simulink model "TorqueVect_HIL_CAN"  (R2022a)
settings: Solver=VariableStepAuto  StartTime=0.0  StopTime=300  RelTol=1e-3
PreLoadFcn:
  | run('Parameters\FSE_Parameters.m')
values from neighbouring files (symbols this model uses):
  Kd = 0;')    [open_carmaker_gui.m]
  Ki = 0    [open_carmaker_gui.m]
undefined symbols (not defined in the file or in its folder): BRegenEnabledButton, canChannel, CyalphaLookUp, efficiency, Fz_curve, Fz_scaling_long, gearR, izz, jw, kd, ki, Kp, kp, l_f, l_r, lambda, m, Mz_max, N, N_lat, N_long, P_max, pid_kd_lat, pid_kd_long, pid_ki_lat, pid_ki_long, pid_kp_lat, pid_kp_long, R_max, rw, steerR, T_i_max, TC_Decr_Gas, TC_Derivative, TC_Incr_Gas, TC_On, TC_Relay_Off, TC_Relay_On, tireCornerStiffness, Ts, TV_On, TV_Override, velocity_lookup, velocity_lookup_lat, y_ref, yrr_scaling
libraries: simulink x218, slpidlib x135, CarMaker4SL x73, TractionControlLibrary x13, canmsglib x11, canlib x10, TorqueVectoringLibrary x6, simulink_extras x4, PedalConversionLibrary x3, PowerControlLibrary x1
(part 4 of 26)

== system TorqueVect_HIL_CAN/CarMaker/IPG Vehicle/PowerTrain/PTControl Example/PTControl_ALL_CTRL_VC_MFE24/New TC ==
  lim 1 : Inport
  lim 2 : Inport  Port=2
  lim 3 : Inport  Port=3
  lim 4 : Inport  Port=4
  vx : Inport  Port=5
  w_FL : Inport  Port=6
  w_FR : Inport  Port=7
  w_RL : Inport  Port=8
  w_RR : Inport  Port=9
  Front SR Target : Inport  Port=10
  Rear SR Target : Inport  Port=11
  P_TC : Inport  Port=12
  D_TC : Inport  Port=13
  enable_tc : Inport  Port=14
  rate_h : Inport  Port=15
  rate_l : Inport  Port=16
  Demux1 : Demux
  Gain : Gain  Gain=0.2032/13.39
  Rate Limiter Dynamic{,1..3} (4 alike) : simulink/Discontinuities/Rate Limiter Dynamic
  Reference Generator1 : Subsystem
  Saturation : Saturate  UpperLimit=inf  LowerLimit=0
  Subtract1 : Sum  Inputs=-+
  TC R1 : Subsystem
  TC R2 : Subsystem
  TC R3 : Subsystem
  TC R4 : Subsystem
  Vector Concatenate3 : Concatenate  NumInputs=4
  R1 Demand : Outport
  L1 Demand : Outport  Port=2
  R2 Demand : Outport  Port=3
  L2 Demand : Outport  Port=4
  wires:
  Reference Generator1/1(R1) -> TC R1/1(modified slip ratio reference)
  lim 1/1 -> TC R1/2(lim 1)
  Gain/1 -> Subtract1/2
  Vector Concatenate3/1 -> Gain/1  "omega"
  Subtract1/1 -> Demux1/1
  vx/1 -> Saturation/1
  TC R2/1(Control Effort 1) -> Rate Limiter Dynamic1/2  "MMotorL1Demand"
  w_RL/1 -> Vector Concatenate3/4
  w_RR/1 -> Vector Concatenate3/3
  w_FL/1 -> Vector Concatenate3/2
  w_FR/1 -> Vector Concatenate3/1
  Front SR Target/1 -> Reference Generator1/2(Front SR Target)
  Rear SR Target/1 -> Reference Generator1/3(Rear SR Target)
  lim 2/1 -> TC R2/2(lim 1)
  lim 3/1 -> TC R3/2(lim 1)
  lim 4/1 -> TC R4/2(lim 1)
  Reference Generator1/2(L1) -> TC R2/1(modified slip ratio reference)
  Reference Generator1/3(R2) -> TC R3/1(modified slip ratio reference)
  Reference Generator1/4(L2) -> TC R4/1(modified slip ratio reference)
  P_TC/1 -> TC R2/4(P_TC), TC R4/4(P_TC), TC R3/4(P_TC), TC R1/4(P_TC)
  D_TC/1 -> TC R2/5(D_TC), TC R4/5(D_TC), TC R3/5(D_TC), TC R1/5(D_TC)
  Demux1/1 -> TC R1/3(modified slip ratio measurement)
  Demux1/2 -> TC R2/3(modified slip ratio measurement)
  Demux1/3 -> TC R3/3(modified slip ratio measurement)
  Demux1/4 -> TC R4/3(modified slip ratio measurement)
  TC R1/1(Control Effort 1) -> Rate Limiter Dynamic/2  "MMotorR1Demand"
  Saturation/1 -> Subtract1/1, Reference Generator1/1(x2)
  TC R3/1(Control Effort 1) -> Rate Limiter Dynamic2/2
  TC R4/1(Control Effort 1) -> Rate Limiter Dynamic3/2
  enable_tc/1 -> TC R4/6(enable_tc), TC R2/6(enable_tc), TC R3/6(enable_tc), TC R1/6(enable_tc)
  Rate Limiter Dynamic/1 -> R1 Demand/1
  rate_h/1 -> Rate Limiter Dynamic3/1, Rate Limiter Dynamic2/1, Rate Limiter Dynamic1/1, Rate Limiter Dynamic/1
  rate_l/1 -> Rate Limiter Dynamic/3, Rate Limiter Dynamic3/3, Rate Limiter Dynamic2/3, Rate Limiter Dynamic1/3
  Rate Limiter Dynamic1/1 -> L1 Demand/1
  Rate Limiter Dynamic2/1 -> R2 Demand/1
  Rate Limiter Dynamic3/1 -> L2 Demand/1

== system TorqueVect_HIL_CAN/CarMaker/IPG Vehicle/PowerTrain/PTControl Example/PTControl_ALL_CTRL_VC_MFE24/PTC ==
  Constant2 : Constant
  Ground : Ground
  Mode_EngineDrive : Constant  Value=4
  Mux : Mux
  OperState_Driving : Constant  Value=4
  PTC MiscOut : Outport  VectorParamsAs1DForOutWhenUnconnected=off
  wires:
  Constant2/1 -> Mux/4  "Ignition"
  Mode_EngineDrive/1 -> Mux/3
  Ground/1 -> Mux/2  "OperationError"
  OperState_Driving/1 -> Mux/1
  Mux/1 -> PTC MiscOut/1

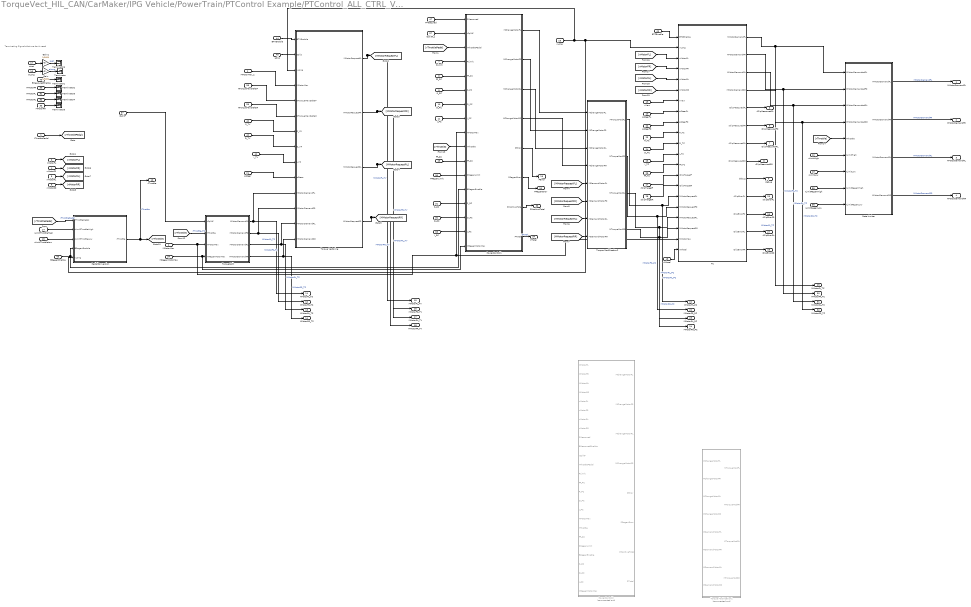
== system TorqueVect_HIL_CAN/CarMaker/IPG Vehicle/PowerTrain/PTControl Example/PTControl_ALL_CTRL_VC_MFE24/Subsystem ==
  note: Terminating Signals that we don't need
  rThrottlePedal : Inport
  MMotorMax : Inport  Port=2
  nMotorFL : Inport  Port=3
  nMotorFR : Inport  Port=4
  nMotorRL : Inport  Port=5
  nMotorRR : Inport  Port=6
  PLimit : Inport  Port=7
  FF_PC : Inport  Port=8
  P_PC : Inport  Port=9
  D_PC : Inport  Port=10
  I_PC : Inport  Port=11
  rLimitHigh : Inport  Port=12
  rLimitLow : Inport  Port=13
  rLimitThrottleHigh : Inport  Port=14
  rLimitThrottleLow : Inport  Port=15
  aLong : Inport  Port=16
  aLat : Inport  Port=17
  vLong : Inport  Port=18
  nYaw : Inport  Port=19
  aSteerFL : Inport  Port=20
  aSteer : Inport  Port=21
  aSteerFR : Inport  Port=22
  P_TC : Inport  Port=23
  D_TC : Inport  Port=24
  I_TC : Inport  Port=25
  FF_TC : Inport  Port=26
  rSlipTargetF : Inport  Port=27
  rSlipTargetR : Inport  Port=28
  FF_RC : Inport  Port=29
  PRegenLimit : Inport  Port=30
  P_RC : Inport  Port=31
  D_RC : Inport  Port=32
  I_RC : Inport  Port=33
  MRegenMotorMax : Inport  Port=34
  rLimitRegenHigh : Inport  Port=35
  rLimitRegenLow : Inport  Port=36
  rSplitF : Inport  Port=37
  NTorqueMaxDeltaF : Inport  Port=38
  NTorqueMaxDeltaR : Inport  Port=39
  P_TV : Inport  Port=40
  I_TV : Inport  Port=41
  D_TV : Inport  Port=42
  BRegenEnable : Inport  Port=43
  BTVEnable : Inport  Port=44
  aSlip : Inport  Port=45
  BTCEnable : Inport  Port=46
  PMeasured : Inport  Port=47  OutMin=-250000  OutMax=250000  Unit=W  PortDimensions=1
      settings: AttributesFormatString=[%<OutMin>, %<OutMax>] %<Unit>
  rWheel : Inport  Port=48
  BMeasuredEnable : Inport  Port=49
  MMotorFR : Inport  Port=50
  MMotorFL : Inport  Port=51
  MMotorRL : Inport  Port=52
  MMotorRR : Inport  Port=53
  Gain : Gain  Gain=1/9.81
  Gain1 : Gain  Gain=1/9.81
  MMotorMax_1 : InportShadow  Port=2
  PedalConversion : Subsystem
  PowerControl1 : Subsystem
  PowerControl2 : Subsystem  Commented=on
  Rate Limiter : Subsystem
  TC : Subsystem
  Terminator{,1..6} (7 alike) : Terminator
  Torque Modification1 : Subsystem  Commented=on
  Torque Modification2 : Subsystem
  Torque Vectoring : Subsystem
  TorqueSplit : Subsystem
  rSplitF_1 : InportShadow  Port=37
  MMotorDemandFL : Outport
  MMotorDemandFR : Outport  Port=2
  MMotorDemandRL : Outport  Port=3
  MMotorDemandRR : Outport  Port=4
  rSlipMeasuredFL : Outport  Port=5
  rSlipMeasuredFR : Outport  Port=6
  rSlipMeasuredRL : Outport  Port=7
  rSlipMeasuredRR : Outport  Port=8
  debug : Outport  Port=9
  rThrottle : Outport  Port=10
  MMotorFL_TS : Outport  Port=11
  MMotorFR_TS : Outport  Port=12
  MMotorRL_TS : Outport  Port=13
  MMotorRR_TS : Outport  Port=14
  MMotorFL_TV : Outport  Port=15
  MMotorFR_TV : Outport  Port=16
  MMotorRL_TV : Outport  Port=17
  MMotorRR_TV : Outport  Port=18
  PError : Outport  Port=19
  PRegenError : Outport  Port=20
  MMotorFL_PC : Outport  Port=21
  MMotorFR_PC : Outport  Port=22
  MMotorRL_PC : Outport  Port=23
  MMotorRR_PC : Outport  Port=24
  rSlipErrorFL : Outport  Port=25
  rSlipErrorFR : Outport  Port=26
  rSlipErrorRL : Outport  Port=27
  rSlipErrorRR : Outport  Port=28
  MMotorFL_TC : Outport  Port=29
  MMotorFR_TC : Outport  Port=30
  MMotorRL_TC : Outport  Port=31
  MMotorRR_TC : Outport  Port=32
  PPositiveTotal : Outport  Port=33
  PTotal : Outport  Port=34
  wires:
  nMotorFR/1 -> [nMotorFR]
  nMotorRR/1 -> [nMotorRR]
  rSlipTargetF/1 -> TC/14(rSlipTargetF)
  Torque Vectoring/1(MMotorRequestFL) -> MMotorFL_TV/1, [MMotorRequestFL]  "MMotorFL_TV"
  nMotorRL/1 -> [nMotorRL]
  P_RC/1 -> PowerControl1/14(P_RC)
  TC/2(MMotorDemandFR) -> MMotorFR_TC/1, Rate Limiter/2(MMotorDemandedFR)  "MMotorFR_TC"
  [nMotorFL] -> TC/3(nMotorFL)
  MRegenMotorMax/1 -> PowerControl1/17(MRegenMotorMax), TorqueSplit/4(MRegenMotorMax)
  Torque Vectoring/4(MMotorRequestRR) -> MMotorRR_TV/1, [MMotorRequestRR]  "MMotorRR_TV"
  PedalConversion/1(rThrottle) -> rThrottle/1, [rThrottle]  "rThrottle"
  rSlipTargetR/1 -> TC/15(rSlipTargetR)
  [rThrottle] -> TorqueSplit/2(rThrottle)  "rThrottle_TS"
  FF_PC/1 -> PowerControl1/5(FF_PC)
  aLong/1 -> Gain/1
  Torque Vectoring/2(MMotorRequestFR) -> MMotorFR_TV/1, [MMotorRequestFR]  "MMotorFR_TV"
  TC/1(MMotorDemandFL) -> MMotorFL_TC/1, Rate Limiter/1(MMotorDemandedFL)  "MMotorFL_TC"
  TC/10(rSlipErrorFL) -> rSlipErrorFL/1
  [rThrottle] -> Rate Limiter/5(rThrottle)
  rLimitThrottleHigh/1 -> PedalConversion/2(rLimitThrottleHigh)
  [MMotorRequestRL] -> Torque Modification2/7(MDemandMotorRL)
  TC/3(MMotorDemandRL) -> Rate Limiter/3(MMotorDemandedRL), MMotorRL_TC/1  "MMotorRL_TC"
  I_TC/1 -> TC/12(I_TC)
  TorqueSplit/2(MMotorDemandFR) -> MMotorFR_TS/1, Torque Vectoring/12(MMotorDemandFR)  "MMotorFR_TS"
  rLimitHigh/1 -> Rate Limiter/6(rLimitHigh)
  TC/5(rSlipMeasuredFL) -> rSlipMeasuredFL/1
  MMotorMax/1 -> PowerControl1/9(MMotorMax), TC/20(MMotorMax), TorqueSplit/3(MMotorMax)
  [nMotorRR] -> TC/6(nMotorRR)
  [rThrottle] -> PowerControl1/10(rThrottle)
  aSteerFR/1 -> TC/9(aSteerFR)
  Torque Vectoring/3(MMotorRequestRL) -> MMotorRL_TV/1, [MMotorRequestRL]  "MMotorRL_TV"
  rLimitRegenHigh/1 -> Rate Limiter/8(rLimitRegenHigh)
  P_TC/1 -> TC/10(P_TC)
  rSplitF/1 -> TorqueSplit/1(rSplitF)
  TorqueSplit/3(MMotorDemandRL) -> MMotorRL_TS/1, Torque Vectoring/13(MMotorDemandRL)  "MMotorRL_TS"
  [MMotorRequestRR] -> Torque Modification2/8(MDemandMotorRR)
  FF_TC/1 -> TC/13(FF_TC)
  P_PC/1 -> PowerControl1/6(P_PC)
  rLimitRegenLow/1 -> Rate Limiter/9(rLimitRegenLow)
  [MMotorRequestFL] -> Torque Modification2/5(MDemandMotorFL)
  [nMotorFR] -> TC/4(nMotorFR)
  rLimitLow/1 -> Rate Limiter/7(rLimitLow)
  D_TC/1 -> TC/11(D_TC)
  D_RC/1 -> PowerControl1/15(D_RC)
  vLong/1 -> Torque Vectoring/3(vLong), TC/2(vLong), PedalConversion/5(vLong)
  nYaw/1 -> TC/7(nYaw)
  TC/6(rSlipMeasuredFR) -> rSlipMeasuredFR/1
  PRegenLimit/1 -> PowerControl1/12(PRegenLimit)
  MMotorMax_1/1 -> Torque Vectoring/4(MMotorMax)
  rLimitThrottleLow/1 -> PedalConversion/3(rLimitThrottleLow)
  Rate Limiter/4(MMotorDemandRR) -> MMotorDemandRR/1  "MMotorDemandRR"
  nMotorFL/1 -> [nMotorFL]
  PLimit/1 -> PowerControl1/4(PLimit)
  Rate Limiter/3(MMotorDemandRL) -> MMotorDemandRL/1  "MMotorDemandRL"
  P_TV/1 -> Torque Vectoring/7(P_YR)
  rThrottlePedal/1 -> [rThrottlePedal]
  NTorqueMaxDeltaF/1 -> Torque Vectoring/5(NTorqueMaxDeltaF)
  rSplitF_1/1 -> PowerControl1/2(rSplitF)
  BTVEnable/1 -> Torque Vectoring/1(BTVEnable)
  TC/9(debug) -> debug/1
  D_TV/1 -> Torque Vectoring/8(D_YR)
  TC/7(rSlipMeasuredRL) -> rSlipMeasuredRL/1
  BTCEnable/1 -> TC/1(BTCEnable)
  [rThrottlePedal] -> PedalConversion/1(rThrottlePedal)  "rThrottlePedal"
  Rate Limiter/2(MMotorDemandFR) -> MMotorDemandFR/1  "MMotorDemandFR"
  TorqueSplit/1(MMotorDemandFL) -> MMotorFL_TS/1, Torque Vectoring/11(MMotorDemandFL)  "MMotorFL_TS"
  NTorqueMaxDeltaR/1 -> Torque Vectoring/6(NTorqueMaxDeltaR)
  TC/13(rSlipErrorRR) -> rSlipErrorRR/1
  aSteerFL/1 -> TC/8(aSteerFL)
  I_TV/1 -> Torque Vectoring/9(I_YR)
  TC/11(rSlipErrorFR) -> rSlipErrorFR/1
  I_RC/1 -> PowerControl1/16(I_RC)
  [MMotorRequestFR] -> Torque Modification2/6(MDemandMotorFR)
  [nMotorRL] -> TC/5(nMotorRL)
  aSlip/1 -> Torque Vectoring/2(aSlip)
  Rate Limiter/1(MMotorDemandFL) -> MMotorDemandFL/1  "MMotorDemandFL"
  I_PC/1 -> PowerControl1/8(I_PC)
  TC/4(MMotorDemandRR) -> MMotorRR_TC/1, Rate Limiter/4(MMotorDemandedRR)  "MMotorRR_TC"
  D_PC/1 -> PowerControl1/7(D_PC)
  [rThrottlePedal] -> PowerControl1/3(rThrottlePedal)
  TC/8(rSlipMeasuredRR) -> rSlipMeasuredRR/1
  BRegenEnable/1 -> PowerControl1/13(BRegenEnable), PedalConversion/4(BRegenEnable)
  TorqueSplit/4(MMotorDemandRR) -> MMotorRR_TS/1, Torque Vectoring/14(MMotorDemandRR)  "MMotorRR_TS"
  TC/12(rSlipErrorRL) -> rSlipErrorRL/1
  PMeasured/1 -> PowerControl1/1(PMeasured)
  rWheel/1 -> TC/21(rWheel)
  PowerControl1/5(PError) -> PError/1
  PowerControl1/6(PRegenError) -> PRegenError/1
  PowerControl1/7(PPositiveTotal) -> PPositiveTotal/1
  Torque Modification2/1(MTorqueModFL) -> MMotorFL_PC/1, TC/16(MMotorRequestFL)  "MMotorFL_PC"
  Torque Modification2/2(MTorqueModFR) -> MMotorFR_PC/1, TC/17(MMotorRequestFR)  "MMotorFR_PC"
  Torque Modification2/3(MTorqueModRL) -> TC/18(MMotorRequestRL), MMotorRL_PC/1  "MMotorRL_PC"
  Torque Modification2/4(MTorqueModRR) -> TC/19(MMotorRequestRR), MMotorRR_PC/1  "MMotorRR_PC"
  FF_RC/1 -> PowerControl1/11(FF_RC)
  BMeasuredEnable/1 -> Terminator1/1
  MMotorRR/1 -> Terminator5/1
  MMotorRL/1 -> Terminator4/1
  MMotorFL/1 -> Terminator3/1
  MMotorFR/1 -> Terminator2/1
  PowerControl1/8(PTotal) -> PTotal/1  "PTotal"
  PowerControl1/1(MChangeMotorFL) -> Torque Modification2/1(MChangeMotorFL)
  PowerControl1/2(MChangeMotorFR) -> Torque Modification2/2(MChangeMotorFR)
  PowerControl1/3(MChangeMotorRL) -> Torque Modification2/3(MChangeMotorRL)
  PowerControl1/4(MChangeMotorRR) -> Torque Modification2/4(MChangeMotorRR)
  Gain/1 -> Terminator/1  "aLong"
  aLat/1 -> Gain1/1
  Gain1/1 -> Terminator6/1  "aLat"
  aSteer/1 -> Torque Vectoring/10(aSteer)

== system TorqueVect_HIL_CAN/CarMaker/IPG Vehicle/PowerTrain/PTControl Example/PTControl_ALL_CTRL_VC_REGEN/New TC ==
  lim 1 : Inport
  lim 2 : Inport  Port=2
  lim 3 : Inport  Port=3
  lim 4 : Inport  Port=4
  vx : Inport  Port=5
  w_FL : Inport  Port=6
  w_FR : Inport  Port=7
  w_RL : Inport  Port=8
  w_RR : Inport  Port=9
  Front SR Target : Inport  Port=10
  Rear SR Target : Inport  Port=11
  P_TC : Inport  Port=12
  D_TC : Inport  Port=13
  enable_tc : Inport  Port=14
  rate_h : Inport  Port=15
  rate_l : Inport  Port=16
  Demux1 : Demux
  Gain : Gain  Gain=0.2032/13.39
  Rate Limiter Dynamic{,1..3} (4 alike) : simulink/Discontinuities/Rate Limiter Dynamic
  Reference Generator1 : Subsystem
  Saturation : Saturate  UpperLimit=inf  LowerLimit=0
  Subtract1 : Sum  Inputs=-+
  TC R1 : Subsystem
  TC R2 : Subsystem
  TC R3 : Subsystem
  TC R4 : Subsystem
  Vector Concatenate3 : Concatenate  NumInputs=4
  R1 Demand : Outport
  L1 Demand : Outport  Port=2
  R2 Demand : Outport  Port=3
  L2 Demand : Outport  Port=4
  wires:
  Reference Generator1/1(R1) -> TC R1/1(modified slip ratio reference)
  lim 1/1 -> TC R1/2(lim 1)
  Gain/1 -> Subtract1/2
  Vector Concatenate3/1 -> Gain/1  "omega"
  Subtract1/1 -> Demux1/1
  vx/1 -> Saturation/1
  TC R2/1(Control Effort 1) -> Rate Limiter Dynamic1/2  "MMotorL1Demand"
  w_RL/1 -> Vector Concatenate3/4
  w_RR/1 -> Vector Concatenate3/3
  w_FL/1 -> Vector Concatenate3/2
  w_FR/1 -> Vector Concatenate3/1
  Front SR Target/1 -> Reference Generator1/2(Front SR Target)
  Rear SR Target/1 -> Reference Generator1/3(Rear SR Target)
  lim 2/1 -> TC R2/2(lim 1)
  lim 3/1 -> TC R3/2(lim 1)
  lim 4/1 -> TC R4/2(lim 1)
  Reference Generator1/2(L1) -> TC R2/1(modified slip ratio reference)
  Reference Generator1/3(R2) -> TC R3/1(modified slip ratio reference)
  Reference Generator1/4(L2) -> TC R4/1(modified slip ratio reference)
  P_TC/1 -> TC R2/4(P_TC), TC R4/4(P_TC), TC R3/4(P_TC), TC R1/4(P_TC)
  D_TC/1 -> TC R2/5(D_TC), TC R4/5(D_TC), TC R3/5(D_TC), TC R1/5(D_TC)
  Demux1/1 -> TC R1/3(modified slip ratio measurement)
  Demux1/2 -> TC R2/3(modified slip ratio measurement)
  Demux1/3 -> TC R3/3(modified slip ratio measurement)
  Demux1/4 -> TC R4/3(modified slip ratio measurement)
  TC R1/1(Control Effort 1) -> Rate Limiter Dynamic/2  "MMotorR1Demand"
  Saturation/1 -> Subtract1/1, Reference Generator1/1(x2)
  TC R3/1(Control Effort 1) -> Rate Limiter Dynamic2/2
  TC R4/1(Control Effort 1) -> Rate Limiter Dynamic3/2
  enable_tc/1 -> TC R4/6(enable_tc), TC R2/6(enable_tc), TC R3/6(enable_tc), TC R1/6(enable_tc)
  Rate Limiter Dynamic/1 -> R1 Demand/1
  rate_h/1 -> Rate Limiter Dynamic3/1, Rate Limiter Dynamic2/1, Rate Limiter Dynamic1/1, Rate Limiter Dynamic/1
  rate_l/1 -> Rate Limiter Dynamic/3, Rate Limiter Dynamic3/3, Rate Limiter Dynamic2/3, Rate Limiter Dynamic1/3
  Rate Limiter Dynamic1/1 -> L1 Demand/1
  Rate Limiter Dynamic2/1 -> R2 Demand/1
  Rate Limiter Dynamic3/1 -> L2 Demand/1

== system TorqueVect_HIL_CAN/CarMaker/IPG Vehicle/PowerTrain/PTControl Example/PTControl_ALL_CTRL_VC_REGEN/PTC ==
  Constant2 : Constant
  Ground : Ground
  Mode_EngineDrive : Constant  Value=4
  Mux : Mux
  OperState_Driving : Constant  Value=4
  PTC MiscOut : Outport  VectorParamsAs1DForOutWhenUnconnected=off
  wires:
  Constant2/1 -> Mux/4  "Ignition"
  Mode_EngineDrive/1 -> Mux/3
  Ground/1 -> Mux/2  "OperationError"
  OperState_Driving/1 -> Mux/1
  Mux/1 -> PTC MiscOut/1

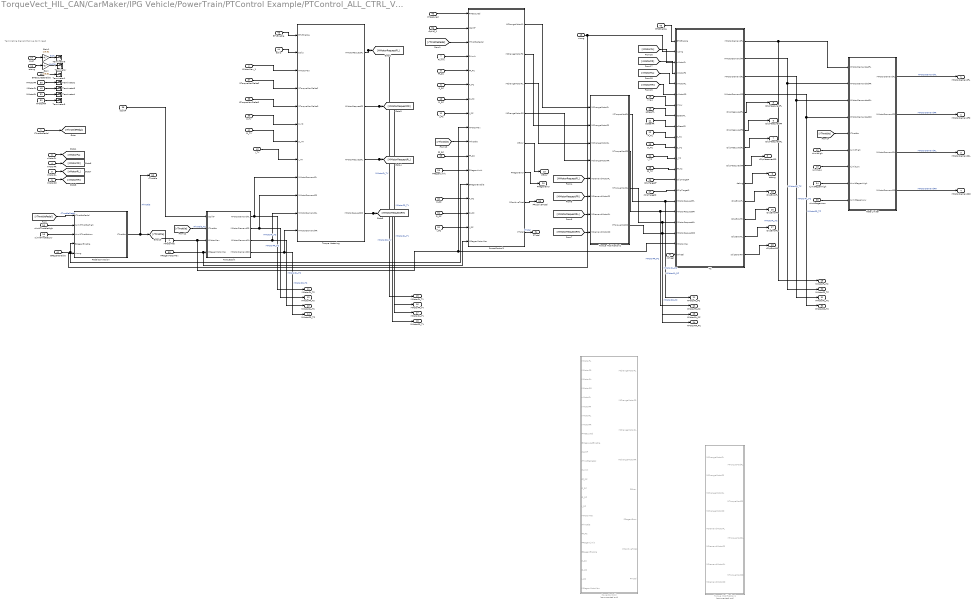
== system TorqueVect_HIL_CAN/CarMaker/IPG Vehicle/PowerTrain/PTControl Example/PTControl_ALL_CTRL_VC_REGEN/Subsystem ==
  note: Terminating Signals that we don't need
  rThrottlePedal : Inport
  MMotorMax : Inport  Port=2
  nMotorFL : Inport  Port=3
  nMotorFR : Inport  Port=4
  nMotorRL : Inport  Port=5
  nMotorRR : Inport  Port=6
  PLimit : Inport  Port=7
  FF_PC : Inport  Port=8
  P_PC : Inport  Port=9
  D_PC : Inport  Port=10
  I_PC : Inport  Port=11
  rLimitHigh : Inport  Port=12
  rLimitLow : Inport  Port=13
  rLimitThrottleHigh : Inport  Port=14
  rLimitThrottleLow : Inport  Port=15
  aLong : Inport  Port=16
  aLat : Inport  Port=17
  vLong : Inport  Port=18
  nYaw : Inport  Port=19
  aSteerFL : Inport  Port=20
  aSteerFR : Inport  Port=21
  P_TC : Inport  Port=22
  D_TC : Inport  Port=23
  I_TC : Inport  Port=24
  FF_TC : Inport  Port=25
  rSlipTargetF : Inport  Port=26
  rSlipTargetR : Inport  Port=27
  FF_RC : Inport  Port=28
  PRegenLimit : Inport  Port=29
  P_RC : Inport  Port=30
  D_RC : Inport  Port=31
  I_RC : Inport  Port=32
  MRegenMotorMax : Inport  Port=33
  rLimitRegenHigh : Inport  Port=34
  rLimitRegenLow : Inport  Port=35
  rSplitF : Inport  Port=36
  NTorqueMaxDeltaF : Inport  Port=37
  NTorqueMaxDeltaR : Inport  Port=38
  P_TV : Inport  Port=39
  I_TV : Inport  Port=40
  D_TV : Inport  Port=41
  BRegenEnable : Inport  Port=42
  BTVEnable : Inport  Port=43
  aSlip : Inport  Port=44
  BTCEnable : Inport  Port=45
  PMeasured : Inport  Port=46  OutMin=-250000  OutMax=250000  Unit=W  PortDimensions=1
      settings: AttributesFormatString=[%<OutMin>, %<OutMax>] %<Unit>
  rWheel : Inport  Port=47
  BMeasuredEnable : Inport  Port=48
  MMotorFL : Inport  Port=49
  MMotorFR : Inport  Port=50
  MMotorRL : Inport  Port=51
  MMotorRR : Inport  Port=52
  Gain : Gain  Gain=1/9.81
  Gain1 : Gain  Gain=1/9.81
  MMotorMax_1 : InportShadow  Port=2
  PedalConversion : Subsystem
  PowerControl1 : Subsystem
  PowerControl2 : Subsystem  Commented=on
  Rate Limiter : Subsystem
  TC : Subsystem
  Terminator{,1..6} (7 alike) : Terminator
  Torque Modification1 : Subsystem  Commented=on
  Torque Modification2 : Subsystem
  Torque Vectoring : Subsystem
  TorqueSplit : Subsystem
  rSplitF_1 : InportShadow  Port=36
  MMotorDemandFL : Outport
  MMotorDemandFR : Outport  Port=2
  MMotorDemandRL : Outport  Port=3
  MMotorDemandRR : Outport  Port=4
  rSlipMeasuredFL : Outport  Port=5
  rSlipMeasuredFR : Outport  Port=6
  rSlipMeasuredRL : Outport  Port=7
  rSlipMeasuredRR : Outport  Port=8
  debug : Outport  Port=9
  rThrottle : Outport  Port=10
  MMotorFL_TS : Outport  Port=11
  MMotorFR_TS : Outport  Port=12
  MMotorRL_TS : Outport  Port=13
  MMotorRR_TS : Outport  Port=14
  MMotorFL_TV : Outport  Port=15
  MMotorFR_TV : Outport  Port=16
  MMotorRL_TV : Outport  Port=17
  MMotorRR_TV : Outport  Port=18
  PError : Outport  Port=19
  PRegenError : Outport  Port=20
  MMotorFL_PC : Outport  Port=21
  MMotorFR_PC : Outport  Port=22
  MMotorRL_PC : Outport  Port=23
  MMotorRR_PC : Outport  Port=24
  rSlipErrorFL : Outport  Port=25
  rSlipErrorFR : Outport  Port=26
  rSlipErrorRL : Outport  Port=27
  rSlipErrorRR : Outport  Port=28
  MMotorFL_TC : Outport  Port=29
  MMotorFR_TC : Outport  Port=30
  MMotorRL_TC : Outport  Port=31
  MMotorRR_TC : Outport  Port=32
  PPositiveTotal : Outport  Port=33
  PTotal : Outport  Port=34
  wires:
  nMotorFR/1 -> [nMotorFR]
  nMotorRR/1 -> [nMotorRR]
  rSlipTargetF/1 -> TC/14(rSlipTargetF)
  Torque Vectoring/1(MMotorRequestFL) -> MMotorFL_TV/1, [MMotorRequestFL]  "MMotorFL_TV"
  nMotorRL/1 -> [nMotorRL]
  P_RC/1 -> PowerControl1/14(P_RC)
  TC/2(MMotorDemandFR) -> MMotorFR_TC/1, Rate Limiter/2(MMotorDemandedFR)  "MMotorFR_TC"
  [nMotorFL] -> TC/3(nMotorFL)
  MRegenMotorMax/1 -> PowerControl1/17(MRegenMotorMax), TorqueSplit/4(MRegenMotorMax)
  Torque Vectoring/4(MMotorRequestRR) -> MMotorRR_TV/1, [MMotorRequestRR]  "MMotorRR_TV"
  PedalConversion/1(rThrottle) -> rThrottle/1, [rThrottle]  "rThrottle"
  rSlipTargetR/1 -> TC/15(rSlipTargetR)
  [rThrottle] -> TorqueSplit/2(rThrottle)  "rThrottle_TS"
  FF_PC/1 -> PowerControl1/5(FF_PC)
  aLong/1 -> Gain/1
  Torque Vectoring/2(MMotorRequestFR) -> MMotorFR_TV/1, [MMotorRequestFR]  "MMotorFR_TV"
  TC/1(MMotorDemandFL) -> MMotorFL_TC/1, Rate Limiter/1(MMotorDemandedFL)  "MMotorFL_TC"
  TC/10(rSlipErrorFL) -> rSlipErrorFL/1
  [rThrottle] -> Rate Limiter/5(rThrottle)
  rLimitThrottleHigh/1 -> PedalConversion/2(rLimitThrottleHigh)
  [MMotorRequestRL] -> Torque Modification2/7(MDemandMotorRL)
  TC/3(MMotorDemandRL) -> Rate Limiter/3(MMotorDemandedRL), MMotorRL_TC/1  "MMotorRL_TC"
  I_TC/1 -> TC/12(I_TC)
  TorqueSplit/2(MMotorDemandFR) -> MMotorFR_TS/1, Torque Vectoring/10(MMotorDemandFR)  "MMotorFR_TS"
  rLimitHigh/1 -> Rate Limiter/6(rLimitHigh)
  TC/5(rSlipMeasuredFL) -> rSlipMeasuredFL/1
  MMotorMax/1 -> PowerControl1/9(MMotorMax), TC/20(MMotorMax), TorqueSplit/3(MMotorMax)
  [nMotorRR] -> TC/6(nMotorRR)
  [rThrottle] -> PowerControl1/10(rThrottle)
  aSteerFR/1 -> TC/9(aSteerFR)
  Torque Vectoring/3(MMotorRequestRL) -> MMotorRL_TV/1, [MMotorRequestRL]  "MMotorRL_TV"
  rLimitRegenHigh/1 -> Rate Limiter/8(rLimitRegenHigh)
  P_TC/1 -> TC/10(P_TC)
  rSplitF/1 -> TorqueSplit/1(rSplitF)
  TorqueSplit/3(MMotorDemandRL) -> MMotorRL_TS/1, Torque Vectoring/11(MMotorDemandRL)  "MMotorRL_TS"
  [MMotorRequestRR] -> Torque Modification2/8(MDemandMotorRR)
  FF_TC/1 -> TC/13(FF_TC)
  P_PC/1 -> PowerControl1/6(P_PC)
  rLimitRegenLow/1 -> Rate Limiter/9(rLimitRegenLow)
  [MMotorRequestFL] -> Torque Modification2/5(MDemandMotorFL)
  [nMotorFR] -> TC/4(nMotorFR)
  rLimitLow/1 -> Rate Limiter/7(rLimitLow)
  D_TC/1 -> TC/11(D_TC)
  D_RC/1 -> PowerControl1/15(D_RC)
  vLong/1 -> TC/2(vLong), PedalConversion/5(vLong)
  nYaw/1 -> TC/7(nYaw)
  TC/6(rSlipMeasuredFR) -> rSlipMeasuredFR/1
  PRegenLimit/1 -> PowerControl1/12(PRegenLimit)
  MMotorMax_1/1 -> Torque Vectoring/3(MMotorMax)
  rLimitThrottleLow/1 -> PedalConversion/3(rLimitThrottleLow)
  Rate Limiter/4(MMotorDemandRR) -> MMotorDemandRR/1  "MMotorDemandRR"
  nMotorFL/1 -> [nMotorFL]
  PLimit/1 -> PowerControl1/4(PLimit)
  Rate Limiter/3(MMotorDemandRL) -> MMotorDemandRL/1  "MMotorDemandRL"
  P_TV/1 -> Torque Vectoring/6(P_YR)
  rThrottlePedal/1 -> [rThrottlePedal]
  NTorqueMaxDeltaF/1 -> Torque Vectoring/4(NTorqueMaxDeltaF)
  rSplitF_1/1 -> PowerControl1/2(rSplitF)
  BTVEnable/1 -> Torque Vectoring/1(BTVEnable)
  TC/9(debug) -> debug/1
  D_TV/1 -> Torque Vectoring/7(D_YR)
  TC/7(rSlipMeasuredRL) -> rSlipMeasuredRL/1
  BTCEnable/1 -> TC/1(BTCEnable)
  [rThrottlePedal] -> PedalConversion/1(rThrottlePedal)  "rThrottlePedal"
  Rate Limiter/2(MMotorDemandFR) -> MMotorDemandFR/1  "MMotorDemandFR"
  TorqueSplit/1(MMotorDemandFL) -> MMotorFL_TS/1, Torque Vectoring/9(MMotorDemandFL)  "MMotorFL_TS"
  NTorqueMaxDeltaR/1 -> Torque Vectoring/5(NTorqueMaxDeltaR)
  TC/13(rSlipErrorRR) -> rSlipErrorRR/1
  aSteerFL/1 -> TC/8(aSteerFL)
  I_TV/1 -> Torque Vectoring/8(I_YR)
  TC/11(rSlipErrorFR) -> rSlipErrorFR/1
  I_RC/1 -> PowerControl1/16(I_RC)
  [MMotorRequestFR] -> Torque Modification2/6(MDemandMotorFR)
  [nMotorRL] -> TC/5(nMotorRL)
  aSlip/1 -> Torque Vectoring/2(aSlip)
  Rate Limiter/1(MMotorDemandFL) -> MMotorDemandFL/1  "MMotorDemandFL"
  I_PC/1 -> PowerControl1/8(I_PC)
  TC/4(MMotorDemandRR) -> MMotorRR_TC/1, Rate Limiter/4(MMotorDemandedRR)  "MMotorRR_TC"
  D_PC/1 -> PowerControl1/7(D_PC)
  [rThrottlePedal] -> PowerControl1/3(rThrottlePedal)
  TC/8(rSlipMeasuredRR) -> rSlipMeasuredRR/1
  BRegenEnable/1 -> PowerControl1/13(BRegenEnable), PedalConversion/4(BRegenEnable)
  TorqueSplit/4(MMotorDemandRR) -> MMotorRR_TS/1, Torque Vectoring/12(MMotorDemandRR)  "MMotorRR_TS"
  TC/12(rSlipErrorRL) -> rSlipErrorRL/1
  PMeasured/1 -> PowerControl1/1(PMeasured)
  rWheel/1 -> TC/21(rWheel)
  PowerControl1/5(PError) -> PError/1
  PowerControl1/6(PRegenError) -> PRegenError/1
  PowerControl1/7(PPositiveTotal) -> PPositiveTotal/1
  Torque Modification2/1(MTorqueModFL) -> MMotorFL_PC/1, TC/16(MMotorRequestFL)  "MMotorFL_PC"
  Torque Modification2/2(MTorqueModFR) -> MMotorFR_PC/1, TC/17(MMotorRequestFR)  "MMotorFR_PC"
  Torque Modification2/3(MTorqueModRL) -> TC/18(MMotorRequestRL), MMotorRL_PC/1  "MMotorRL_PC"
  Torque Modification2/4(MTorqueModRR) -> TC/19(MMotorRequestRR), MMotorRR_PC/1  "MMotorRR_PC"
  FF_RC/1 -> PowerControl1/11(FF_RC)
  BMeasuredEnable/1 -> Terminator1/1
  MMotorRR/1 -> Terminator5/1
  MMotorRL/1 -> Terminator4/1
  MMotorFL/1 -> Terminator3/1
  MMotorFR/1 -> Terminator2/1
  PowerControl1/8(PTotal) -> PTotal/1  "PTotal"
  PowerControl1/1(MChangeMotorFL) -> Torque Modification2/1(MChangeMotorFL)
  PowerControl1/2(MChangeMotorFR) -> Torque Modification2/2(MChangeMotorFR)
  PowerControl1/3(MChangeMotorRL) -> Torque Modification2/3(MChangeMotorRL)
  PowerControl1/4(MChangeMotorRR) -> Torque Modification2/4(MChangeMotorRR)
  Gain/1 -> Terminator/1  "aLong"
  aLat/1 -> Gain1/1
  Gain1/1 -> Terminator6/1  "aLat"

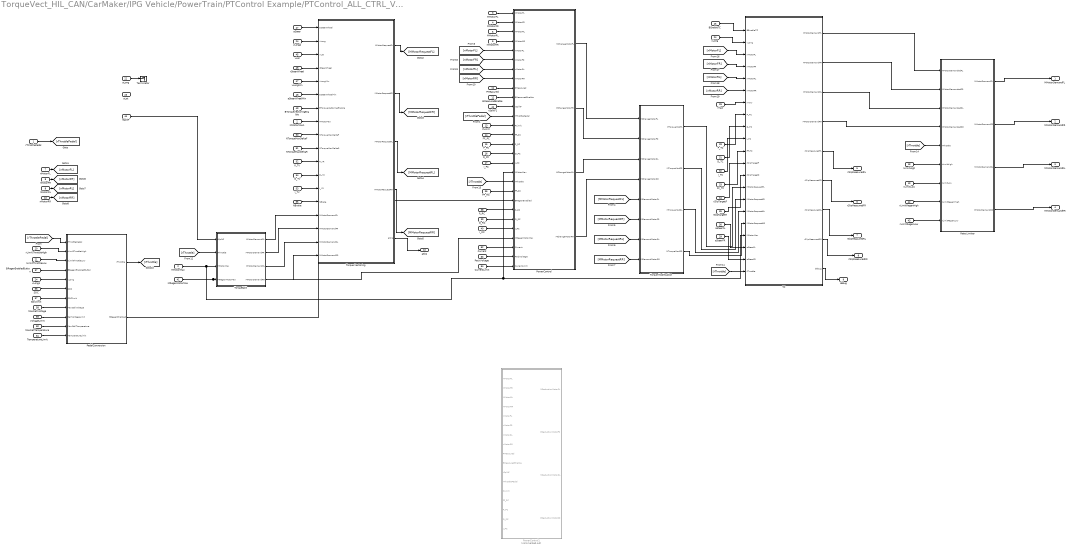
== system TorqueVect_HIL_CAN/CarMaker/IPG Vehicle/PowerTrain/PTControl Example/PTControl_ALL_CTRL_VC_REGEN/Subsystem1 ==
  rThrottlePedal : Inport
  MMotorMax : Inport  Port=2
  MMotorFL : Inport  Port=3
  MMotorFR : Inport  Port=4
  MMotorRL : Inport  Port=5
  MMotorRR : Inport  Port=6
  nMotorFL : Inport  Port=7
  nMotorFR : Inport  Port=8
  nMotorRL : Inport  Port=9
  nMotorRR : Inport  Port=10
  PMeasured : Inport  Port=11
  BMeasuredEnable : Inport  Port=12
  PLimit : Inport  Port=13
  FF_PC : Inport  Port=14
  P_PC : Inport  Port=15
  D_PC : Inport  Port=16
  I_PC : Inport  Port=17
  rLimitHigh : Inport  Port=18
  rLimitLow : Inport  Port=19
  rLimitThrottleHigh : Inport  Port=20
  rLimitThrottleLow : Inport  Port=21
  aLong : Inport  Port=22
  aLat : Inport  Port=23
  vLong : Inport  Port=24
  BEnableTC : Inport  Port=25
  nYaw : Inport  Port=26
  aSteer : Inport  Port=27
  P_TC : Inport  Port=28
  aSteerFR : Inport  Port=29
  aSteerFL : Inport  Port=30
  D_TC : Inport  Port=31
  I_TC : Inport  Port=32
  FF_TC : Inport  Port=33
  rSlipTargetF : Inport  Port=34
  rSlipTargetR : Inport  Port=35
  FF_RC : Inport  Port=36
  BRegenEnabledButton : Inport  Port=37
  P_RC : Inport  Port=38
  D_RC : Inport  Port=39
  I_RC : Inport  Port=40
  MRegenMotorMax : Inport  Port=41
  rLimitRegenHigh : Inport  Port=42
  rLimitRegenLow : Inport  Port=43
  rSplitF : Inport  Port=44
  vLat : Inport  Port=45
  rSteerWheel : Inport  Port=46
  vLongMin : Inport  Port=47
  aSteerWheelMin : Inport  Port=48
  BTorqueVectoringEnable : Inport  Port=49
  NTorqueMaxDeltaF : Inport  Port=50
  NTorqueMaxDeltaR : Inport  Port=51
  P_TV : Inport  Port=52
  I_TV : Inport  Port=53
  D_TV : Inport  Port=54
  NBrake : Inport  Port=55
  SOC : Inport  Port=56
  SOClimit : Inport  Port=57
  MaxCellVoltage : Inport  Port=58
  VoltageLimit : Inport  Port=59
  MaxCellTemperature : Inport  Port=60
  TemperatureLimit : Inport  Port=61
  Current : Inport  Port=62
  PackVoltage : Inport  Port=63
  CurrentLimit : Inport  Port=64
  MMotorMax1 : InportShadow  Port=2
  PedalConversion : Subsystem
  PowerControl : Subsystem
  PowerControl1 : Subsystem  Commented=on
  Rate Limiter : Subsystem
  TC : Subsystem
  Terminator : Terminator
  Torque Modification : Subsystem
  Torque Vectoring : Subsystem
  TorqueSplit : Subsystem
  rSplitF1 : InportShadow  Port=44
  vLong1 : InportShadow  Port=24
  vLong2 : InportShadow  Port=24
  MMotorDemandFL : Outport
  MMotorDemandFR : Outport  Port=2
  MMotorDemandRL : Outport  Port=3
  MMotorDemandRR : Outport  Port=4
  rSlipMeasuredFL : Outport  Port=5
  rSlipMeasuredFR : Outport  Port=6
  rSlipMeasuredRL : Outport  Port=7
  rSlipMeasuredRR : Outport  Port=8
  debug : Outport  Port=9
  aSlip : Outport  Port=10
  wires:
  FF_PC/1 -> PowerControl/14(FF_PC)
  MMotorFR/1 -> PowerControl/2(MMotorFR)
  P_PC/1 -> PowerControl/15(P_PC)
  rThrottlePedal/1 -> [rThrottlePedal]
  MMotorFL/1 -> PowerControl/1(MMotorFL)
  PLimit/1 -> PowerControl/13(PLimit)
  PedalConversion/1(rThrottle) -> [rThrottle]
  D_PC/1 -> PowerControl/16(D_PC)
  [rThrottlePedal] -> PowerControl/12(rThrottlePedal)
  I_PC/1 -> PowerControl/17(I_PC)
  MMotorRR/1 -> PowerControl/4(MMotorRR)
  MMotorRL/1 -> PowerControl/3(MMotorRL)
  PMeasured/1 -> PowerControl/9(PMeasured)
  BMeasuredEnable/1 -> PowerControl/10(BMeasuredEnable)
  [rThrottlePedal] -> PedalConversion/1(rThrottlePedal)
  Rate Limiter/1(MMotorDemandFL) -> MMotorDemandFL/1
  Rate Limiter/2(MMotorDemandFR) -> MMotorDemandFR/1
  Rate Limiter/3(MMotorDemandRL) -> MMotorDemandRL/1
  Rate Limiter/4(MMotorDemandRR) -> MMotorDemandRR/1
  rLimitHigh/1 -> Rate Limiter/6(rLimitHigh)
  rSplitF/1 -> TorqueSplit/1(rSplitF)
  MMotorMax/1 -> TC/18(MMotorMax), PowerControl/18(MMotorMax), TorqueSplit/3(MMotorMax)
  rLimitThrottleHigh/1 -> PedalConversion/2(rLimitThrottleHigh)
  rLimitThrottleLow/1 -> PedalConversion/3(rLimitThrottleLow)
  [nMotorFR] -> TC/4(nMotorFR)
  [nMotorFL] -> TC/3(nMotorFL)
  [nMotorRL] -> TC/5(nMotorRL)
  rSlipTargetR/1 -> TC/13(rSlipTargetR)
  P_TC/1 -> TC/8(P_TC)
  rSlipTargetF/1 -> TC/12(rSlipTargetF)
  [nMotorRR] -> TC/6(nMotorRR)
  BEnableTC/1 -> TC/1(BEnableTC)
  I_TC/1 -> TC/10(I_TC)
  D_TC/1 -> TC/9(D_TC)
  FF_TC/1 -> TC/11(FF_TC)
  nYaw/1 -> TC/7(nYaw)
  nMotorFL/1 -> [nMotorFL]
  nMotorFR/1 -> [nMotorFR]
  nMotorRL/1 -> [nMotorRL]
  nMotorRR/1 -> [nMotorRR]
  [nMotorRR] -> PowerControl/8(nMotorRR)
  [nMotorRL] -> PowerControl/7(nMotorRL)
  [nMotorFR] -> PowerControl/6(nMotorFR)
  [nMotorFL] -> PowerControl/5(nMotorFL)
  PowerControl/1(MChangeMotorFL) -> Torque Modification/1(MChangeMotorFL)
  PowerControl/2(MChangeMotorFR) -> Torque Modification/2(MChangeMotorFR)
  PowerControl/3(MChangeMotorRL) -> Torque Modification/3(MChangeMotorRL)
  PowerControl/4(MChangeMotorRR) -> Torque Modification/4(MChangeMotorRR)
  [MMotorRequestFL] -> Torque Modification/5(MDemandMotorFL)
  [MMotorRequestFR] -> Torque Modification/6(MDemandMotorFR)
  [MMotorRequestRL] -> Torque Modification/7(MDemandMotorRL)
  [MMotorRequestRR] -> Torque Modification/8(MDemandMotorRR)
  Torque Modification/4(MTorqueModRR) -> TC/17(MMotorRequestRR)
  Torque Modification/3(MTorqueModRL) -> TC/16(MMotorRequestRL)
  Torque Modification/2(MTorqueModFR) -> TC/15(MMotorRequestFR)
  Torque Modification/1(MTorqueModFL) -> TC/14(MMotorRequestFL)
  TC/1(MMotorDemandFL) -> Rate Limiter/1(MMotorDemandedFL)
  TC/2(MMotorDemandFR) -> Rate Limiter/2(MMotorDemandedFR)
  TC/3(MMotorDemandRL) -> Rate Limiter/3(MMotorDemandedRL)
  TC/4(MMotorDemandRR) -> Rate Limiter/4(MMotorDemandedRR)
  aLong/1 -> Terminator/1
  TC/5(rSlipMeasuredFL) -> rSlipMeasuredFL/1
  TC/6(rSlipMeasuredFR) -> rSlipMeasuredFR/1
  TC/7(rSlipMeasuredRL) -> rSlipMeasuredRL/1
  TC/8(rSlipMeasuredRR) -> rSlipMeasuredRR/1
  TC/9(debug) -> debug/1
  FF_RC/1 -> PowerControl/20(FF_RC)
  vLong1/1 -> PedalConversion/5(vLong)
  BRegenEnabledButton/1 -> PedalConversion/4(BRegenEnabledButton)
  P_RC/1 -> PowerControl/22(P_RC)
  D_RC/1 -> PowerControl/23(D_RC)
  I_RC/1 -> PowerControl/24(I_RC)
  MRegenMotorMax/1 -> PowerControl/25(MRegenMotorMax), TorqueSplit/4(MRegenMotorMax)
  [rThrottle] -> TorqueSplit/2(rThrottle)
  [rThrottle] -> PowerControl/19(rThrottle)
  [rThrottle] -> Rate Limiter/5(rThrottle)
  rLimitRegenHigh/1 -> Rate Limiter/8(rLimitRegenHigh)
  vLong/1 -> TC/2(vLong)
  rLimitLow/1 -> Rate Limiter/7(rLimitLow)
  rLimitRegenLow/1 -> Rate Limiter/9(rLimitRegenLow)
  Torque Vectoring/1(MMotorRequestFL) -> [MMotorRequestFL]
  Torque Vectoring/2(MMotorRequestFR) -> [MMotorRequestFR]
  Torque Vectoring/3(MMotorRequestRL) -> [MMotorRequestRL]
  Torque Vectoring/4(MMotorRequestRR) -> [MMotorRequestRR]
  TorqueSplit/1(MMotorDemandFL) -> Torque Vectoring/15(MMotorDemandFL)
  TorqueSplit/2(MMotorDemandFR) -> Torque Vectoring/16(MMotorDemandFR)
  TorqueSplit/3(MMotorDemandRL) -> Torque Vectoring/17(MMotorDemandRL)
  TorqueSplit/4(MMotorDemandRR) -> Torque Vectoring/18(MMotorDemandRR)
  aSteer/1 -> Torque Vectoring/1(aSteerWheel)
  vLong2/1 -> Torque Vectoring/2(vLong)
  vLat/1 -> Torque Vectoring/3(vLat)
  rSteerWheel/1 -> Torque Vectoring/4(rSteerWheel)
  vLongMin/1 -> Torque Vectoring/5(vLongMin)
  aSteerWheelMin/1 -> Torque Vectoring/6(aSteerWheelMin)
  BTorqueVectoringEnable/1 -> Torque Vectoring/7(BTorqueVectoringEnable)
  MMotorMax1/1 -> Torque Vectoring/8(MMotorMax)
  NTorqueMaxDeltaF/1 -> Torque Vectoring/9(NTorqueMaxDeltaF)
  NTorqueMaxDeltaR/1 -> Torque Vectoring/10(NTorqueMaxDeltaR)
  P_TV/1 -> Torque Vectoring/11(P_YR)
  I_TV/1 -> Torque Vectoring/13(I_YR)
  D_TV/1 -> Torque Vectoring/12(D_YR)
  NBrake/1 -> Torque Vectoring/14(NBrake)
  rSplitF1/1 -> PowerControl/11(rSplitF)
  PedalConversion/2(BRegenEnabled) -> PowerControl/21(BRegenEnabled)
  SOC/1 -> PedalConversion/6(SOC)
  SOClimit/1 -> PedalConversion/7(SOClimit)
  TemperatureLimit/1 -> PedalConversion/11(TemperatureLimit)
  MaxCellVoltage/1 -> PedalConversion/8(MaxCellVoltage)
  MaxCellTemperature/1 -> PedalConversion/10(MaxCellTemperature)
  VoltageLimit/1 -> PedalConversion/9(CellVoltageLimit)
  PackVoltage/1 -> PowerControl/27(PackVoltage)
  Current/1 -> PowerControl/26(Current)
  CurrentLimit/1 -> PowerControl/28(CurrentLimit)
  Torque Vectoring/5(aSlip) -> aSlip/1
  [rThrottle] -> TC/21(rThrottle)
  aSteerFL/1 -> TC/19(aSteerFL)
  aSteerFR/1 -> TC/20(aSteerFR)

== system TorqueVect_HIL_CAN/CarMaker/IPG Vehicle/PowerTrain/PTControl Example/PTControl_ALL_Speedgoat/New TC ==
  lim 1 : Inport
  lim 2 : Inport  Port=2
  lim 3 : Inport  Port=3
  lim 4 : Inport  Port=4
  vx : Inport  Port=5
  w_FL : Inport  Port=6
  w_FR : Inport  Port=7
  w_RL : Inport  Port=8
  w_RR : Inport  Port=9
  Front SR Target : Inport  Port=10
  Rear SR Target : Inport  Port=11
  P_TC : Inport  Port=12
  D_TC : Inport  Port=13
  enable_tc : Inport  Port=14
  rate_h : Inport  Port=15
  rate_l : Inport  Port=16
  Demux1 : Demux
  Gain : Gain  Gain=0.2032/13.39
  Rate Limiter Dynamic{,1..3} (4 alike) : simulink/Discontinuities/Rate Limiter Dynamic
  Reference Generator1 : Subsystem
  Saturation : Saturate  UpperLimit=inf  LowerLimit=0
  Subtract1 : Sum  Inputs=-+
  TC R1 : Subsystem
  TC R2 : Subsystem
  TC R3 : Subsystem
  TC R4 : Subsystem
  Vector Concatenate3 : Concatenate  NumInputs=4
  R1 Demand : Outport
  L1 Demand : Outport  Port=2
  R2 Demand : Outport  Port=3
  L2 Demand : Outport  Port=4
  wires:
  Reference Generator1/1(R1) -> TC R1/1(modified slip ratio reference)
  lim 1/1 -> TC R1/2(lim 1)
  Gain/1 -> Subtract1/2
  Vector Concatenate3/1 -> Gain/1  "omega"
  Subtract1/1 -> Demux1/1
  vx/1 -> Saturation/1
  TC R2/1(Control Effort 1) -> Rate Limiter Dynamic1/2  "MMotorL1Demand"
  w_RL/1 -> Vector Concatenate3/4
  w_RR/1 -> Vector Concatenate3/3
  w_FL/1 -> Vector Concatenate3/2
  w_FR/1 -> Vector Concatenate3/1
  Front SR Target/1 -> Reference Generator1/2(Front SR Target)
  Rear SR Target/1 -> Reference Generator1/3(Rear SR Target)
  lim 2/1 -> TC R2/2(lim 1)
  lim 3/1 -> TC R3/2(lim 1)
  lim 4/1 -> TC R4/2(lim 1)
  Reference Generator1/2(L1) -> TC R2/1(modified slip ratio reference)
  Reference Generator1/3(R2) -> TC R3/1(modified slip ratio reference)
  Reference Generator1/4(L2) -> TC R4/1(modified slip ratio reference)
  P_TC/1 -> TC R2/4(P_TC), TC R4/4(P_TC), TC R3/4(P_TC), TC R1/4(P_TC)
  D_TC/1 -> TC R2/5(D_TC), TC R4/5(D_TC), TC R3/5(D_TC), TC R1/5(D_TC)
  Demux1/1 -> TC R1/3(modified slip ratio measurement)
  Demux1/2 -> TC R2/3(modified slip ratio measurement)
  Demux1/3 -> TC R3/3(modified slip ratio measurement)
  Demux1/4 -> TC R4/3(modified slip ratio measurement)
  TC R1/1(Control Effort 1) -> Rate Limiter Dynamic/2  "MMotorR1Demand"
  Saturation/1 -> Subtract1/1, Reference Generator1/1(x2)
  TC R3/1(Control Effort 1) -> Rate Limiter Dynamic2/2
  TC R4/1(Control Effort 1) -> Rate Limiter Dynamic3/2
  enable_tc/1 -> TC R4/6(enable_tc), TC R2/6(enable_tc), TC R3/6(enable_tc), TC R1/6(enable_tc)
  Rate Limiter Dynamic/1 -> R1 Demand/1
  rate_h/1 -> Rate Limiter Dynamic3/1, Rate Limiter Dynamic2/1, Rate Limiter Dynamic1/1, Rate Limiter Dynamic/1
  rate_l/1 -> Rate Limiter Dynamic/3, Rate Limiter Dynamic3/3, Rate Limiter Dynamic2/3, Rate Limiter Dynamic1/3
  Rate Limiter Dynamic1/1 -> L1 Demand/1
  Rate Limiter Dynamic2/1 -> R2 Demand/1
  Rate Limiter Dynamic3/1 -> L2 Demand/1

== system TorqueVect_HIL_CAN/CarMaker/IPG Vehicle/PowerTrain/PTControl Example/PTControl_ALL_Speedgoat/PTC ==
  Constant2 : Constant
  Ground : Ground
  Mode_EngineDrive : Constant  Value=4
  Mux : Mux
  OperState_Driving : Constant  Value=4
  PTC MiscOut : Outport  VectorParamsAs1DForOutWhenUnconnected=off
  wires:
  Constant2/1 -> Mux/4  "Ignition"
  Mode_EngineDrive/1 -> Mux/3
  Ground/1 -> Mux/2  "OperationError"
  OperState_Driving/1 -> Mux/1
  Mux/1 -> PTC MiscOut/1

== system TorqueVect_HIL_CAN/CarMaker/IPG Vehicle/PowerTrain/PTControl Example/PTControl_ALL_Speedgoat/Subsystem ==
  VhclCtrl.PT : Inport
  PTControl_In : Inport  Port=2
  Bus Selector : BusSelector  OutputSignals=VhclCtrl Gas,VhclCtrl Brake
  Bus Selector1 : BusSelector  OutputSignals=Vel_B x,Vel_B y,Omega_B z,Acc_B x,Acc_B y
  Bus Selector2 : BusSelector  OutputSignals=PT:Motor.PT:Motor:Trq,PT:Motor.PT:Motor1:Trq,PT:Motor.PT:Motor2:Trq,PT:Motor.PT:Motor3:Trq,PT:Motor.PT:Motor:rotv,PT:Motor.PT:Motor1:rotv,PT:Motor.PT:Motor2:rotv,PT:Motor.PT:Motor3:rotv,Steer.Driver:Steer:Ang,Steer.Car:SteerAngle:FL,Steer.Car:SteerAngle:FR,PT:PwrSupply:HV1:Pwr
  CAN Configuration : canlib/CAN Configuration  BlockHandle=5539.0005  Device=MathWorks Virtual 1 (Channel 1)  DeviceMenu=MathWorks Virtual 1 (Channel 1)  ObjConstructor=canChannel('MathWorks', 'Virtual 1', 1)  BusSpeed=500000  EnableBitParameters=off  AckMode=Normal
      settings: SourceProductBaseCode=VN
  CAN Pack1 : canmsglib/CAN Pack  MsgList=(none)  MsgName=Wheel Torques  MsgIDType=Standard (11-bit identifier)  MsgIdentifier=600  MsgLength=8  Remote=off  ApplyMinMax=off  BusOutput=off  SignalInfo={ 'FL_Trq', '0', '16', 'LE', 'signed', 'Standard', '0', '1', '0', '-210', '210'; 'FR_Trq', '16', '16', 'LE', 'signed', 'Standard', '0', '1', '0', '-210', '210'; 'RL_Trq', '32', '16', 'LE', 'signed', 'Standard', '0', '1', '0', '-210', '210'; 'RR_Trq', '48', '16', 'LE', 'signed', 'Standard', '0', '1', '0', '-210', '210' }
      settings: SourceProductBaseCode=XP,ME,VN  DataFormat=manually specified signals
  CAN Pack2 : canmsglib/CAN Pack  MsgList=(none)  MsgName=Motor Speeds (rad/s)  MsgIDType=Standard (11-bit identifier)  MsgIdentifier=601  MsgLength=8  Remote=off  ApplyMinMax=off  BusOutput=off  SignalInfo={ 'FL_w', '0', '16', 'LE', 'signed', 'Standard', '0', '1', '0', '-32768', '32767'; 'FR_w', '16', '16', 'LE', 'signed', 'Standard', '0', '1', '0', '-32768', '32767'; 'RL_w', '32', '16', 'LE', 'signed', 'Standard', '0', '1', '0', '-32768', '32767'; 'RR_w', '48', '16', 'LE', 'signed', 'Standard', '0', '1', '0', '-32768', '32767' }
      settings: SourceProductBaseCode=XP,ME,VN  DataFormat=manually specified signals
  CAN Pack3 : canmsglib/CAN Pack  MsgList=(none)  MsgName=CAN Msg  MsgIDType=Standard (11-bit identifier)  MsgIdentifier=602  MsgLength=8  Remote=off  ApplyMinMax=off  BusOutput=off  SignalInfo={ 'Throttle', '0', '8', 'LE', 'unsigned', 'Standard', '0', '1', '0', '0', '100'; 'Brake', '8', '8', 'LE', 'unsigned', 'Standard', '0', '1', '0', '0', '100'; 'Steering Angle', '16', '16', 'LE', 'signed', 'Standard', '0', '1', '0', '-32768', '32767'; 'FL Angle', '32', '16', 'LE', 'signed', 'Standard', '0', '1', '0', '-32768', '32767'; 'FR Angle', '48', '16', 'LE', 'signed', 'Standard', '0', '1', '0', '-32768', '32767' }
      settings: SourceProductBaseCode=XP,ME,VN  DataFormat=manually specified signals
  CAN Pack4 : canmsglib/CAN Pack  MsgList=(none)  MsgName=CAN Msg  MsgIDType=Standard (11-bit identifier)  MsgIdentifier=603  MsgLength=8  Remote=off  ApplyMinMax=off  BusOutput=off  SignalInfo={ 'Vx', '0', '16', 'LE', 'signed', 'Standard', '0', '1', '0', '-32768', '32767'; 'Vy', '16', '16', 'LE', 'signed', 'Standard', '0', '1', '0', '-32768', '32767'; 'nYaw', '32', '16', 'LE', 'signed', 'Standard', '0', '1', '0', '-32768', '32767'; 'Power', '48', '16', 'LE', 'signed', 'Standard', '0', '1', '0', '-8000', '8000' }
      settings: SourceProductBaseCode=XP,ME,VN  DataFormat=manually specified signals
  CAN Pack5 : canmsglib/CAN Pack  Commented=on  MsgList=(none)  MsgName=CAN Msg  MsgIDType=Standard (11-bit identifier)  MsgIdentifier=605  MsgLength=8  Remote=off  ApplyMinMax=off  BusOutput=off  SignalInfo={ 'Pwr', '0', '32', 'LE', 'signed', 'Standard', '0', '1', '0', '-Inf', 'Inf' }
      settings: SourceProductBaseCode=XP,ME,VN  DataFormat=manually specified signals
  CAN Pack6 : canmsglib/CAN Pack  MsgList=(none)  MsgName=CAN Msg  MsgIDType=Standard (11-bit identifier)  MsgIdentifier=604  MsgLength=4  Remote=off  ApplyMinMax=off  BusOutput=off  SignalInfo={ 'Ax', '0', '16', 'LE', 'signed', 'Standard', '0', '1', '0', '-32768', '32767'; 'Ay', '16', '16', 'LE', 'signed', 'Standard', '0', '1', '0', '-32768', '32767' }
      settings: SourceProductBaseCode=XP,ME,VN  DataFormat=manually specified signals
  CAN Transmit1 : canlib/CAN Transmit  BlockHandle=5572.0005  Device=MathWorks Virtual 1 (Channel 1)  DeviceMenu=MathWorks Virtual 1 (Channel 1)  ObjConstructor=canChannel('MathWorks', 'Virtual 1', 1)  EnableEventTransmit=off  EnablePeriodicTransmit=on  MessagePeriod=0.01
      settings: SourceProductBaseCode=VN
  CAN Transmit2 : canlib/CAN Transmit  BlockHandle=5574.0005  Device=MathWorks Virtual 1 (Channel 1)  DeviceMenu=MathWorks Virtual 1 (Channel 1)  ObjConstructor=canChannel('MathWorks', 'Virtual 1', 1)  EnableEventTransmit=off  EnablePeriodicTransmit=on  MessagePeriod=0.01
      settings: SourceProductBaseCode=VN
  CAN Transmit3 : canlib/CAN Transmit  BlockHandle=5576.0005  Device=MathWorks Virtual 1 (Channel 1)  DeviceMenu=MathWorks Virtual 1 (Channel 1)  ObjConstructor=canChannel('MathWorks', 'Virtual 1', 1)  EnableEventTransmit=off  EnablePeriodicTransmit=on  MessagePeriod=0.01
      settings: SourceProductBaseCode=VN
  CAN Transmit4 : canlib/CAN Transmit  Commented=on  BlockHandle=5578.0005  Device=MathWorks Virtual 1 (Channel 1)  DeviceMenu=MathWorks Virtual 1 (Channel 1)  ObjConstructor=canChannel('MathWorks', 'Virtual 1', 1)  EnableEventTransmit=off  EnablePeriodicTransmit=on  MessagePeriod=0.01
      settings: SourceProductBaseCode=VN
  CAN Transmit5 : canlib/CAN Transmit  BlockHandle=5580.0005  Device=MathWorks Virtual 1 (Channel 1)  DeviceMenu=MathWorks Virtual 1 (Channel 1)  ObjConstructor=canChannel('MathWorks', 'Virtual 1', 1)  EnableEventTransmit=off  EnablePeriodicTransmit=on  MessagePeriod=0.01
      settings: SourceProductBaseCode=VN
  CAN Transmit6 : canlib/CAN Transmit  BlockHandle=5582.0005  Device=MathWorks Virtual 1 (Channel 1)  DeviceMenu=MathWorks Virtual 1 (Channel 1)  ObjConstructor=canChannel('MathWorks', 'Virtual 1', 1)  EnableEventTransmit=off  EnablePeriodicTransmit=on  MessagePeriod=0.01
      settings: SourceProductBaseCode=VN
  Gain{,1..3} (4 alike) : Gain  Gain=10
  Gain10 : Gain  Gain=1000
  Gain11 : Gain  Gain=1000
  Gain12 : Gain  Gain=1000
  Gain{8..9,13..15,17..18} (7 alike) : Gain  Gain=100
  Gain16 : Gain  Gain=1/10
  Gain{4..7} (4 alike) : Gain  Gain=30/pi
  Inertial Sensor : CarMaker4SL/Sensors/Inertial Sensor  xname=Param_B00  xstime=Continuous
      settings: SourceProductName=CarMaker4SL
  Rate Transition{,1..18} (19 alike) : RateTransition  OutPortSampleTime=0.001
  Subsystem : Subsystem
  Terminator : Terminator
  <PT:Motor:Trq> : Outport
  <PT:Motor1:Trq> : Outport  Port=2
  <PT:Motor2:Trq> : Outport  Port=3
  <PT:Motor3:Trq> : Outport  Port=4
  wires:
  Inertial Sensor/1 -> Terminator/1
  Inertial Sensor/2 -> Bus Selector1/1
  PTControl_In/1 -> Bus Selector2/1
  VhclCtrl.PT/1 -> Bus Selector/1
  Bus Selector2/1 -> Rate Transition/1  "<PT:Motor:Trq>"
  Bus Selector2/2 -> Rate Transition1/1  "<PT:Motor1:Trq>"
  Bus Selector2/3 -> Rate Transition2/1  "<PT:Motor2:Trq>"
  Bus Selector2/4 -> Rate Transition3/1  "<PT:Motor3:Trq>"
  Bus Selector2/5 -> Rate Transition4/1  "<PT:Motor:rotv>"
  Bus Selector2/6 -> Rate Transition5/1  "<PT:Motor1:rotv>"
  Bus Selector2/7 -> Rate Transition6/1  "<PT:Motor2:rotv>"
  Bus Selector2/8 -> Rate Transition7/1  "<PT:Motor3:rotv>"
  Bus Selector/2 -> Rate Transition9/1  "<VhclCtrl Brake>"
  Bus Selector2/9 -> Rate Transition10/1  "<Driver:Steer:Ang>"
  Bus Selector2/10 -> Rate Transition11/1  "<Car:SteerAngle:FL>"
  Bus Selector2/11 -> Rate Transition12/1  "<Car:SteerAngle:FR>"
  Bus Selector1/1 -> Rate Transition14/1  "<Vel_B x>"
  Bus Selector1/2 -> Rate Transition15/1  "<Vel_B y>"
  Bus Selector1/3 -> Rate Transition16/1  "<Omega_B z>"
  Bus Selector2/12 -> Rate Transition13/1  "<PT:PwrSupply:HV1:Pwr>"
  CAN Pack1/1 -> CAN Transmit1/1
  CAN Pack2/1 -> CAN Transmit2/1
  CAN Pack3/1 -> CAN Transmit3/1
  CAN Pack5/1 -> CAN Transmit4/1
  CAN Pack4/1 -> CAN Transmit5/1
  Subsystem/1(Out1) -> <PT:Motor:Trq>/1
  Subsystem/2(Out2) -> <PT:Motor1:Trq>/1
  Subsystem/3(Out3) -> <PT:Motor2:Trq>/1
  Subsystem/4(Out4) -> <PT:Motor3:Trq>/1
  Rate Transition/1 -> Gain/1
  Rate Transition1/1 -> Gain1/1
  Rate Transition2/1 -> Gain2/1
  Rate Transition3/1 -> Gain3/1
  Rate Transition4/1 -> Gain4/1
  Rate Transition5/1 -> Gain5/1
  Rate Transition6/1 -> Gain6/1
  Rate Transition7/1 -> Gain7/1
  Rate Transition9/1 -> Gain9/1
  Rate Transition10/1 -> Gain10/1
  Rate Transition11/1 -> Gain11/1
  Rate Transition12/1 -> Gain12/1
  Rate Transition13/1 -> Gain16/1
  Rate Transition14/1 -> Gain13/1
  Rate Transition15/1 -> Gain14/1
  Rate Transition16/1 -> Gain15/1
  Bus Selector/1 -> Rate Transition8/1  "<VhclCtrl Gas>"
  Rate Transition8/1 -> Gain8/1
  Gain/1 -> CAN Pack1/1
  Gain1/1 -> CAN Pack1/2
  Gain2/1 -> CAN Pack1/3
  Gain3/1 -> CAN Pack1/4
  Gain6/1 -> CAN Pack2/3
  Gain5/1 -> CAN Pack2/2
  Gain7/1 -> CAN Pack2/4
  Gain4/1 -> CAN Pack2/1
  Gain8/1 -> CAN Pack3/1
  Gain9/1 -> CAN Pack3/2
  Gain10/1 -> CAN Pack3/3
  Gain11/1 -> CAN Pack3/4
  Gain12/1 -> CAN Pack3/5
  Gain13/1 -> CAN Pack4/1
  Gain14/1 -> CAN Pack4/2
  Gain15/1 -> CAN Pack4/3
  Gain16/1 -> CAN Pack4/4, CAN Pack5/1
  Bus Selector1/5 -> Rate Transition18/1  "<Acc_B y>"
  Rate Transition18/1 -> Gain17/1
  Rate Transition17/1 -> Gain18/1
  Gain17/1 -> CAN Pack6/2
  Gain18/1 -> CAN Pack6/1
  Bus Selector1/4 -> Rate Transition17/1  "<Acc_B x>"
  CAN Pack6/1 -> CAN Transmit6/1

== system TorqueVect_HIL_CAN/CarMaker/IPG Vehicle/PowerTrain/PTControl Example/PTControl_In1/CreateBus PTC Battery ==
  In : Inport
  BusCreator : BusCreator  Inputs=14
  Demux : Demux  Outputs=14
      settings: DisplayOption=none
  Out : Outport  VectorParamsAs1DForOutWhenUnconnected=off
  wires:
  In/1 -> Demux/1
  BusCreator/1 -> Out/1
  Demux/1 -> BusCreator/1  "PTC BattLVIn SOC"
  Demux/2 -> BusCreator/2  "PTC BattLVIn SOH"
  Demux/3 -> BusCreator/3  "PTC BattLVIn Current"
  Demux/4 -> BusCreator/4  "PTC BattLVIn AOC"
  Demux/5 -> BusCreator/5  "PTC BattLVIn Temp"
  Demux/6 -> BusCreator/6  "PTC BattLVIn Energy"
  Demux/7 -> BusCreator/7  "PTC BattLVIn Pwr_max"
  Demux/8 -> BusCreator/8  "PTC BattHVIn SOC"
  Demux/9 -> BusCreator/9  "PTC BattHVIn SOH"
  Demux/10 -> BusCreator/10  "PTC BattHVIn Current"
  Demux/11 -> BusCreator/11  "PTC BattHVIn AOC"
  Demux/12 -> BusCreator/12  "PTC BattHVIn Temp"
  Demux/13 -> BusCreator/13  "PTC BattHVIn Energy"
  Demux/14 -> BusCreator/14  "PTC BattHVIn Pwr_max"

== system TorqueVect_HIL_CAN/CarMaker/IPG Vehicle/PowerTrain/PTControl Example/PTControl_In1/CreateBus PTC ClutchIn ==
  In : Inport
  BusCreator : BusCreator  Inputs=6
  Demux : Demux  Outputs=6
      settings: DisplayOption=none
  Out : Outport  VectorParamsAs1DForOutWhenUnconnected=off
  wires:
  In/1 -> Demux/1
  BusCreator/1 -> Out/1
  Demux/1 -> BusCreator/1  "PTC ClutchIn Pos"
  Demux/2 -> BusCreator/2  "PTC ClutchIn rotv_in"
  Demux/3 -> BusCreator/3  "PTC ClutchIn rotv_out"
  Demux/4 -> BusCreator/4  "PTC ClutchIn Trq_in"
  Demux/5 -> BusCreator/5  "PTC ClutchIn Trq_out"
  Demux/6 -> BusCreator/6  "PTC ClutchIn i_TrqIn2Out"

== system TorqueVect_HIL_CAN/CarMaker/IPG Vehicle/PowerTrain/PTControl Example/PTControl_In1/CreateBus PTC Control Units ==
  In : Inport
  BusCreator : BusCreator  Inputs=4
  Demux : Demux
      settings: DisplayOption=none
  Out : Outport  VectorParamsAs1DForOutWhenUnconnected=off
  wires:
  In/1 -> Demux/1
  BusCreator/1 -> Out/1
  Demux/1 -> BusCreator/1  "PTC ECU_Status"
  Demux/2 -> BusCreator/2  "PTC MCU_Status"
  Demux/3 -> BusCreator/3  "PTC TCU_Status"
  Demux/4 -> BusCreator/4  "PTC BCU_Status"
